simulink model "wheelspeed"  (Simulink 6.1)
settings: Solver=ode45  StartTime=0.0  StopTime=50  RelTol=1e-3
values from neighbouring files (symbols this model uses):
  alpha = 1/2    (= 0.5)    [parameter_setup.m]
  R = 0.09    [parameter_setup.m]
  theta1 = FrontAngle    (= 35)    [parameter_setup.m]
  theta2 = 180-FrontAngle    (= 145)    [parameter_setup.m]
  theta3 = 180+BackAngle    (= 225)    [parameter_setup.m]
  theta4 = 360-BackAngle    (= 315)    [parameter_setup.m]
  wheel_radius = 0.0254    [parameter_setup.m]
undefined symbols (not defined in the file or in its folder): M
settings Model: Creator=~Alim~  LastModifiedBy=Binaryblade
settings OptimizationCC: InlineInvariantSignals=off
settings DebuggingCC: SignalResolutionControl=UseLocalSettings  SolverPrmCheckMsg=warning  MultiTaskDSMMsg=error
settings GRTTargetCC: TargetFcnLib=ansi_tfl_table_tmw.mat

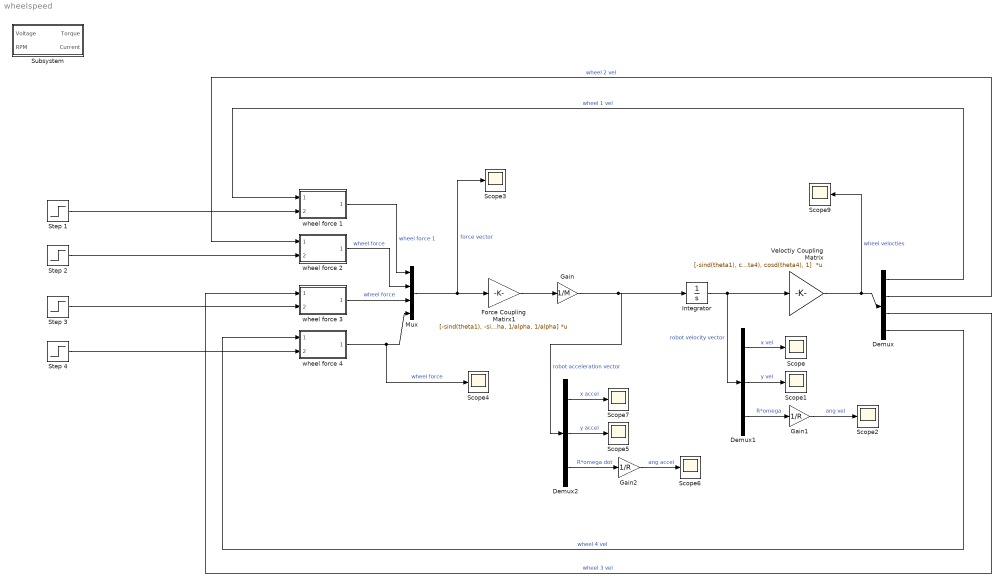
== system wheelspeed ==
  Demux : Demux
  Demux1 : Demux  Outputs=3
  Demux2 : Demux  Outputs=3
  Force Coupling Matirx1 : Gain  Gain=[-sind(theta1), -sind(theta2), -sind(theta3), -sind(theta4); cosd(theta1), cosd(theta2), cosd(theta3), cosd(theta4); 1/alpha, 1/alpha, 1/alpha, 1/alpha]  Multiplication=Matrix(K*u)
  Gain : Gain  Gain=1/M
  Gain1 : Gain  Gain=1/R
  Gain2 : Gain  Gain=1/R
  Integrator : Integrator
  Mux : Mux
  Scope{,1..7,9} (9 alike) : Scope
      Scope2 settings: SaveName=ScopeData2
      Scope3 settings: SaveName=ScopeData3
      Scope4 settings: SaveName=ScopeData4
      Scope5 settings: SaveName=ScopeData5
      Scope6 settings: SaveName=ScopeData6
      Scope7 settings: SaveName=ScopeData7
      Scope9 settings: SaveName=ScopeData9
  Step {1..4} (4 alike) : Step  After=12  SampleTime=0
  Subsystem : Subsystem
  Veloctiy Coupling Matrix : Gain  Gain=[-sind(theta1), cosd(theta1), 1; -sind(theta2), cosd(theta2), 1; -sind(theta3), cosd(theta3), 1; -sind(theta4), cosd(theta4), 1]  Multiplication=Matrix(K*u)
  wheel force 1 : Subsystem
  wheel force 2 : Subsystem
  wheel force 3 : Subsystem
  wheel force 4 : Subsystem
  wires:
  Veloctiy Coupling Matrix/1 -> Demux/1, Scope9/1  "wheel velocties"
  Force Coupling Matirx1/1 -> Gain/1
  Mux/1 -> Force Coupling Matirx1/1, Scope3/1  "force vector"
  Integrator/1 -> Demux1/1, Veloctiy Coupling Matrix/1  "robot velocity vector"
  wheel force 1/1(wheel force) -> Mux/1  "wheel force 1"
  Gain/1 -> Integrator/1, Demux2/1  "robot acceleration vector"
  wheel force 4/1(wheel force) -> Mux/4, Scope4/1  "wheel force"
  wheel force 2/1(wheel force) -> Mux/2  "wheel force"
  wheel force 3/1(wheel force) -> Mux/3  "wheel force"
  Demux1/1 -> Scope/1  "x vel"
  Demux1/2 -> Scope1/1  "y vel"
  Demux1/3 -> Gain1/1  "R*omega"
  Gain1/1 -> Scope2/1  "ang vel"
  Demux2/1 -> Scope7/1  "x accel"
  Demux2/2 -> Scope5/1  "y accel"
  Demux2/3 -> Gain2/1  "R*omega dot"
  Gain2/1 -> Scope6/1  "ang accel"
  Demux/1 -> wheel force 1/1(wheel velocity)  "wheel 1 vel"
  Demux/2 -> wheel force 2/1(wheel velocity)  "wheel 2 vel"
  Demux/3 -> wheel force 3/1(wheel velocity)  "wheel 3 vel"
  Step 1/1 -> wheel force 1/2(voltage)
  Demux/4 -> wheel force 4/1(wheel velocity)  "wheel 4 vel"
  Step 3/1 -> wheel force 3/2(voltage)
  Step 4/1 -> wheel force 4/2(voltage)
  Step 2/1 -> wheel force 2/2(voltage)

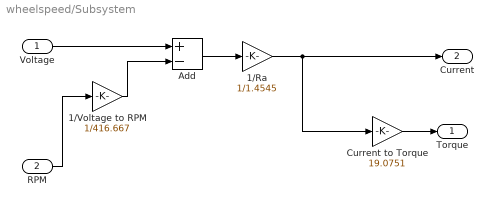
== system wheelspeed/Subsystem ==
  Voltage : Inport  Port=1  LatchInput=off
  RPM : Inport  Port=2  LatchInput=off
  1/Ra : Gain  Gain=1/1.4545
  1/Voltage to RPM : Gain  Gain=1/416.667
  Add : Sum  Inputs=+-  OutScaling=2^-10
  Current to Torque : Gain  Gain=19.0751
  Torque : Outport
  Current : Outport  Port=2
  wires:
  Voltage/1 -> Add/1
  1/Voltage to RPM/1 -> Add/2
  RPM/1 -> 1/Voltage to RPM/1
  Add/1 -> 1/Ra/1
  1/Ra/1 -> Current/1, Current to Torque/1
  Current to Torque/1 -> Torque/1

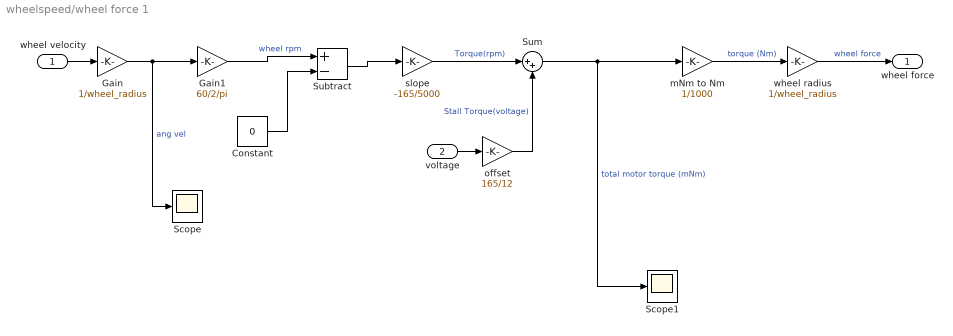
== system wheelspeed/wheel force 1 ==
  wheel velocity : Inport  Port=1  OutDataType=fixdt(1,16,0)  OutScaling=[]  LatchInput=off
  voltage : Inport  Port=2  OutDataType=fixdt(1,16,0)  OutScaling=[]  LatchInput=off
  Constant : Constant  Value=0
  Gain : Gain  Gain=1/wheel_radius
  Gain1 : Gain  Gain=60/2/pi
  Scope : Scope
      settings: SaveName=ScopeData8
  Scope1 : Scope
      settings: SaveName=ScopeData11
  Subtract : Sum  Inputs=+-  OutScaling=2^-10
  Sum : Sum  Inputs=|++
  mNm to Nm : Gain  Gain=1/1000
  offset : Gain  Gain=165/12
  slope : Gain  Gain=-165/5000
  wheel radius : Gain  Gain=1/wheel_radius
  wheel force : Outport  OutDataType=fixdt(1,16,0)  OutScaling=[]
  wires:
  slope/1 -> Sum/1  "Torque(rpm)"
  Sum/1 -> mNm to Nm/1, Scope1/1  "total motor torque (mNm)"
  mNm to Nm/1 -> wheel radius/1  "torque (Nm)"
  Gain/1 -> Gain1/1, Scope/1  "ang vel"
  wheel velocity/1 -> Gain/1
  wheel radius/1 -> wheel force/1  "wheel force"
  voltage/1 -> offset/1
  Constant/1 -> Subtract/2
  Gain1/1 -> Subtract/1  "wheel rpm"
  Subtract/1 -> slope/1
  offset/1 -> Sum/2  "Stall Torque(voltage)"

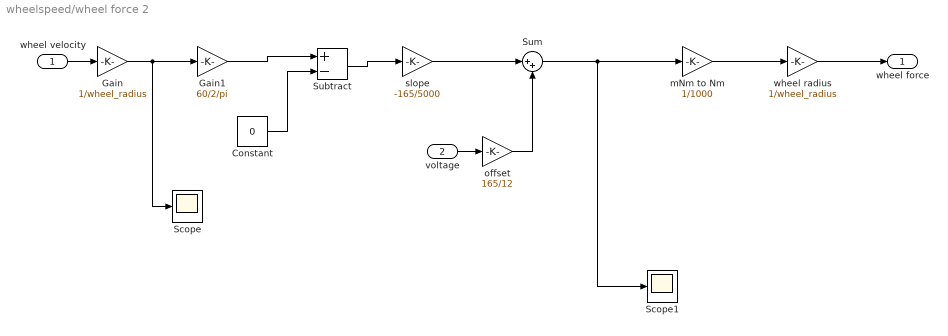
== system wheelspeed/wheel force 2 ==
  wheel velocity : Inport  Port=1  OutDataType=fixdt(1,16,0)  OutScaling=[]  LatchInput=off
  voltage : Inport  Port=2  OutDataType=fixdt(1,16,0)  OutScaling=[]  LatchInput=off
  Constant : Constant  Value=0  VectorParams1D=off
  Gain : Gain  Gain=1/wheel_radius
  Gain1 : Gain  Gain=60/2/pi
  Scope : Scope
      settings: SaveName=ScopeData15
  Scope1 : Scope
      settings: SaveName=ScopeData16
  Subtract : Sum  Inputs=+-  OutScaling=2^-10
  Sum : Sum  Inputs=|++
  mNm to Nm : Gain  Gain=1/1000
  offset : Gain  Gain=165/12
  slope : Gain  Gain=-165/5000
  wheel radius : Gain  Gain=1/wheel_radius
  wheel force : Outport  OutDataType=fixdt(1,16,0)  OutScaling=[]
  wires:
  slope/1 -> Sum/1
  Sum/1 -> Scope1/1, mNm to Nm/1
  mNm to Nm/1 -> wheel radius/1
  Gain/1 -> Scope/1, Gain1/1
  wheel velocity/1 -> Gain/1
  wheel radius/1 -> wheel force/1
  voltage/1 -> offset/1
  Constant/1 -> Subtract/2
  Gain1/1 -> Subtract/1
  Subtract/1 -> slope/1
  offset/1 -> Sum/2

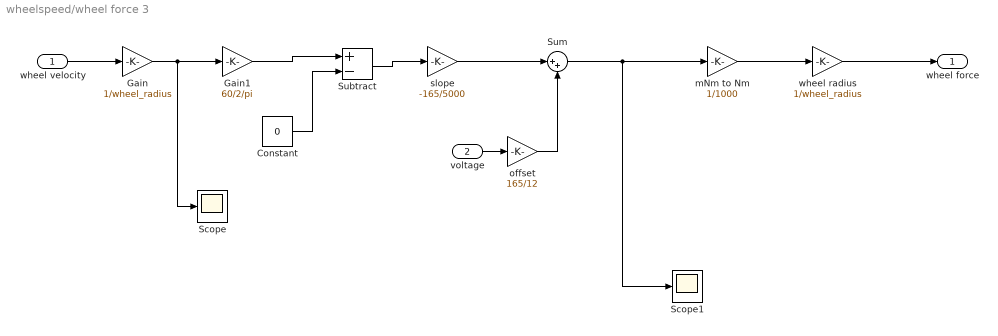
== system wheelspeed/wheel force 3 ==
  wheel velocity : Inport  Port=1  OutDataType=fixdt(1,16,0)  OutScaling=[]  LatchInput=off
  voltage : Inport  Port=2  OutDataType=fixdt(1,16,0)  OutScaling=[]  LatchInput=off
  Constant : Constant  Value=0
  Gain : Gain  Gain=1/wheel_radius
  Gain1 : Gain  Gain=60/2/pi
  Scope : Scope
      settings: SaveName=ScopeData12
  Scope1 : Scope
      settings: SaveName=ScopeData13
  Subtract : Sum  Inputs=+-  OutScaling=2^-10
  Sum : Sum  Inputs=|++
  mNm to Nm : Gain  Gain=1/1000
  offset : Gain  Gain=165/12
  slope : Gain  Gain=-165/5000
  wheel radius : Gain  Gain=1/wheel_radius
  wheel force : Outport  OutDataType=fixdt(1,16,0)  OutScaling=[]
  wires:
  slope/1 -> Sum/1
  Sum/1 -> Scope1/1, mNm to Nm/1
  mNm to Nm/1 -> wheel radius/1
  Gain/1 -> Scope/1, Gain1/1
  voltage/1 -> offset/1
  Constant/1 -> Subtract/2
  Gain1/1 -> Subtract/1
  Subtract/1 -> slope/1
  offset/1 -> Sum/2
  wheel velocity/1 -> Gain/1
  wheel radius/1 -> wheel force/1

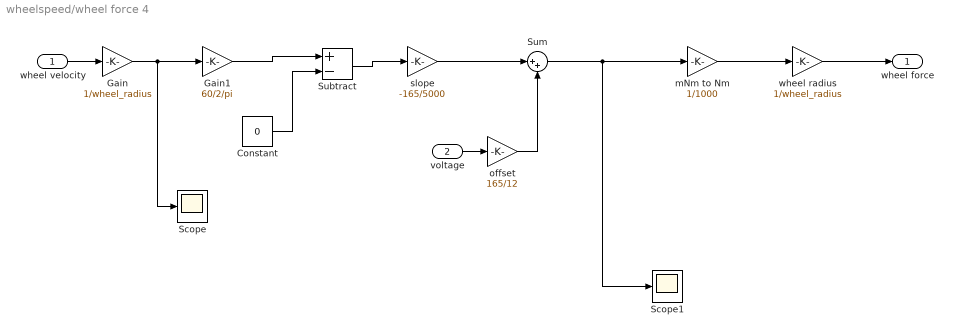
== system wheelspeed/wheel force 4 ==
  wheel velocity : Inport  Port=1  OutDataType=fixdt(1,16,0)  OutScaling=[]  LatchInput=off
  voltage : Inport  Port=2  OutDataType=fixdt(1,16,0)  OutScaling=[]  LatchInput=off
  Constant : Constant  Value=0
  Gain : Gain  Gain=1/wheel_radius
  Gain1 : Gain  Gain=60/2/pi
  Scope : Scope
      settings: SaveName=ScopeData10
  Scope1 : Scope
      settings: SaveName=ScopeData14
  Subtract : Sum  Inputs=+-  OutScaling=2^-10
  Sum : Sum  Inputs=|++
  mNm to Nm : Gain  Gain=1/1000
  offset : Gain  Gain=165/12
  slope : Gain  Gain=-165/5000
  wheel radius : Gain  Gain=1/wheel_radius
  wheel force : Outport  OutDataType=fixdt(1,16,0)  OutScaling=[]
  wires:
  slope/1 -> Sum/1
  Sum/1 -> Scope1/1, mNm to Nm/1
  mNm to Nm/1 -> wheel radius/1
  Gain/1 -> Scope/1, Gain1/1
  wheel velocity/1 -> Gain/1
  wheel radius/1 -> wheel force/1
  voltage/1 -> offset/1
  Constant/1 -> Subtract/2
  Gain1/1 -> Subtract/1
  Subtract/1 -> slope/1
  offset/1 -> Sum/2
